simulink model "iwave_dsa_1ant"  (R2019a)
settings: Solver=VariableStepAuto  StartTime=0.0  StopTime=10.0  RelTol=1e-3
undefined symbols (not defined in the file): i
libraries: xbsIndex_r4 x9262, casper_library_misc x249, xps_library x3, casper_library_reorder x2, casper_library_delays x2
(part 32 of 96)

== system iwave_dsa_1ant/pipeline0/input/bit_stats/histogram ==
  note: pulse extend allows
      | input to AND gate at
      | t + 2^bitwidth + 1
  note: write on t+8, t+9
  note: input valid t+7, t+8
  note: addr presented here
      | t+5, t+6
  note: high t+4, t+5
  note: goes high
      | t+4
  note: new_acc goes high
      | at time t
  note: goes to zero
      | at t + 1
  note: 2^bitwidth extend
      | output goes low
      | at t+(2^bitwidth) + 1
  note: addr input to bram
      | t+6, t+7
  note: capture data 2 of 4 clocks,
      | starting two clocks after new_acc
  note: write on t+8, t+9
  note: goes to zero
      | at t + 1
  note: goes high at
      | at t + 2
  din : Inport
  new_acc : Inport  Port=2
  AddSub1 : xbsIndex_r4/AddSub  mode=Addition  use_carryin=off  use_carryout=off  en=off  latency=1  precision=User Defined  arith_type=Unsigned  n_bits=16  bin_pt=0  quantization=Truncate  overflow=Wrap  use_behavioral_HDL=on  hw_selection=Fabric  pipelined=off  dbl_ovrd=off  block_type=addsub
  AddSub2 : xbsIndex_r4/AddSub  mode=Addition  use_carryin=off  use_carryout=off  en=off  latency=1  precision=User Defined  arith_type=Unsigned  n_bits=16  bin_pt=0  quantization=Truncate  overflow=Wrap  use_behavioral_HDL=on  hw_selection=Fabric  pipelined=off  dbl_ovrd=off  block_type=addsub
  Concat : xbsIndex_r4/Concat  num_inputs=2  dbl_ovrd=off  block_type=concat
  Concat1 : xbsIndex_r4/Concat  num_inputs=2  dbl_ovrd=off  block_type=concat
  Constant1 : xbsIndex_r4/Constant  const=1  gui_display_data_type=Fixed-point  arith_type=Unsigned  n_bits=2  bin_pt=0  preci_type=Single  exp_width=8  frac_width=24  explicit_period=on  period=1  equ=P=C  opselect=C  inp2=PCIN>>17  opr=+  inp1=P  carry=CIN  dbl_ovrd=off  block_type=constant
  Constant2 : xbsIndex_r4/Constant  const=1  gui_display_data_type=Fixed-point  arith_type=Unsigned  n_bits=2  bin_pt=0  preci_type=Single  exp_width=8  frac_width=24  explicit_period=on  period=1  equ=P=C  opselect=C  inp2=PCIN>>17  opr=+  inp1=P  carry=CIN  dbl_ovrd=off  block_type=constant
  Constant3 : xbsIndex_r4/Constant  const=2  gui_display_data_type=Fixed-point  arith_type=Unsigned  n_bits=2  bin_pt=0  preci_type=Single  exp_width=8  frac_width=24  explicit_period=on  period=1  equ=P=C  opselect=C  inp2=PCIN>>17  opr=+  inp1=P  carry=CIN  dbl_ovrd=off  block_type=constant
  Constant4 : xbsIndex_r4/Constant  const=2  gui_display_data_type=Fixed-point  arith_type=Unsigned  n_bits=2  bin_pt=0  preci_type=Single  exp_width=8  frac_width=24  explicit_period=on  period=1  equ=P=C  opselect=C  inp2=PCIN>>17  opr=+  inp1=P  carry=CIN  dbl_ovrd=off  block_type=constant
  Constant5 : xbsIndex_r4/Constant  const=0  gui_display_data_type=Fixed-point  arith_type=Unsigned  n_bits=16  bin_pt=0  preci_type=Single  exp_width=8  frac_width=24  explicit_period=on  period=1  equ=P=C  opselect=C  inp2=PCIN>>17  opr=+  inp1=P  carry=CIN  dbl_ovrd=off  block_type=constant
  Constant6 : xbsIndex_r4/Constant  const=0  gui_display_data_type=Fixed-point  arith_type=Unsigned  n_bits=16  bin_pt=0  preci_type=Single  exp_width=8  frac_width=24  explicit_period=on  period=1  equ=P=C  opselect=C  inp2=PCIN>>17  opr=+  inp1=P  carry=CIN  dbl_ovrd=off  block_type=constant
  Constant7 : xbsIndex_r4/Constant  const=0  gui_display_data_type=Fixed-point  arith_type=Unsigned  n_bits=1  bin_pt=0  preci_type=Single  exp_width=8  frac_width=24  explicit_period=on  period=1  equ=P=C  opselect=C  inp2=PCIN>>17  opr=+  inp1=P  carry=CIN  dbl_ovrd=off  block_type=constant
  Constant8 : xbsIndex_r4/Constant  const=1  gui_display_data_type=Fixed-point  arith_type=Unsigned  n_bits=1  bin_pt=0  preci_type=Single  exp_width=8  frac_width=24  explicit_period=on  period=1  equ=P=C  opselect=C  inp2=PCIN>>17  opr=+  inp1=P  carry=CIN  dbl_ovrd=off  block_type=constant
  Counter1 : xbsIndex_r4/Counter  cnt_type=Free Running  cnt_to=Inf  operation=Up  start_count=0  cnt_by_val=1  arith_type=Unsigned  n_bits=2  bin_pt=0  load_pin=off  rst=on  en=off  explicit_period=on  period=1  use_behavioral_HDL=off  implementation=Fabric  dbl_ovrd=off  block_type=counter
  Counter3 : xbsIndex_r4/Counter  cnt_type=Free Running  cnt_to=Inf  operation=Up  start_count=0  cnt_by_val=1  arith_type=Unsigned  n_bits=bitwidth  bin_pt=0  load_pin=off  rst=off  en=off  explicit_period=on  period=1  use_behavioral_HDL=off  implementation=Fabric  dbl_ovrd=off  block_type=counter
  Counter4 : xbsIndex_r4/Counter  cnt_type=Free Running  cnt_to=Inf  operation=Up  start_count=0  cnt_by_val=1  arith_type=Unsigned  n_bits=2  bin_pt=0  load_pin=off  rst=on  en=off  explicit_period=on  period=1  use_behavioral_HDL=off  implementation=Fabric  dbl_ovrd=off  block_type=counter
  Delay{1..3,5,7..11,13,16..18,20..21,25..27} (18 alike) : xbsIndex_r4/Delay  rst=off  infoeditControl=Selection of Reset will increase slice count due to use of real FFs and instead of SRLs  en=off  latency=1  reg_retiming=off  dbl_ovrd=off  block_type=delay
  Delay{6,12,19,22} (4 alike) : xbsIndex_r4/Delay  rst=off  infoeditControl=Selection of Reset will increase slice count due to use of real FFs and instead of SRLs  en=off  latency=2  reg_retiming=off  dbl_ovrd=off  block_type=delay
  Delay{4,14..15,23} (4 alike) : xbsIndex_r4/Delay  rst=off  infoeditControl=Selection of Reset will increase slice count due to use of real FFs and instead of SRLs  en=off  latency=3  reg_retiming=off  dbl_ovrd=off  block_type=delay
  Delay24 : xbsIndex_r4/Delay  rst=off  infoeditControl=Selection of Reset will increase slice count due to use of real FFs and instead of SRLs  en=off  latency=2^bitwidth  reg_retiming=off  dbl_ovrd=off  block_type=delay
  Delay28 : xbsIndex_r4/Delay  rst=off  infoeditControl=Selection of Reset will increase slice count due to use of real FFs and instead of SRLs  en=off  latency=2^bitwidth  reg_retiming=off  dbl_ovrd=off  block_type=delay
  Delay29 : xbsIndex_r4/Delay  rst=off  infoeditControl=Selection of Reset will increase slice count due to use of real FFs and instead of SRLs  en=off  latency=2^bitwidth  reg_retiming=off  dbl_ovrd=off  block_type=delay
  Gateway Out{1..6} (6 alike) : xbsIndex_r4/Gateway Out  inherit_from_input=off  hdl_port=off  rows=1  columns=1  UseAsDAC=off  DACChannel='1'  interface=None  automatic_assignment=on  address_offset=hex2dec('00')  intf_name=''  intf_description=''  timing_constraint=None  locs_specified=off  LOCs={}  io_standard={}  block_type=gatewayout
  Inverter{,1..4} (5 alike) : xbsIndex_r4/Inverter  en=off  latency=0  dbl_ovrd=off  block_type=inv
  Logical{,2,5,7} (4 alike) : xbsIndex_r4/Logical  logical_function=AND  inputs=2  en=off  latency=1  precision=Full  arith_type=Unsigned  n_bits=16  bin_pt=0  align_bp=on  dbl_ovrd=off  block_type=logical
  Logical{1,3..4,6} (4 alike) : xbsIndex_r4/Logical  logical_function=AND  inputs=2  en=off  latency=0  precision=Full  arith_type=Unsigned  n_bits=16  bin_pt=0  align_bp=on  dbl_ovrd=off  block_type=logical
  Logical8 : xbsIndex_r4/Logical  logical_function=OR  inputs=2  en=off  latency=1  precision=Full  arith_type=Unsigned  n_bits=16  bin_pt=0  align_bp=on  dbl_ovrd=off  block_type=logical
  Mux{,1..5} (6 alike) : xbsIndex_r4/Mux  inputs=2  en=off  latency=1  precision=Full  arith_type=Unsigned  n_bits=16  bin_pt=14  quantization=Truncate  overflow=Wrap  dbl_ovrd=off  block_type=mux
  Register : xbsIndex_r4/Register  init=0  rst=off  en=on  dbl_ovrd=off  block_type=register
  Register1 : xbsIndex_r4/Register  init=0  rst=off  en=on  dbl_ovrd=off  block_type=register
  Relational : xbsIndex_r4/Relational  mode=a=b  op_type=Bool  en=off  latency=0  dbl_ovrd=off  block_type=relational
  Relational1 : xbsIndex_r4/Relational  mode=a=b  op_type=Bool  en=off  latency=0  dbl_ovrd=off  block_type=relational
  Slice : xbsIndex_r4/Slice  nbits=1  boolean_output=on  mode=Lower Bit Location + Width  bit1=0  base1=MSB of Input  bit0=1  base0=LSB of Input  dbl_ovrd=off  block_type=slice
  Slice1 : xbsIndex_r4/Slice  nbits=1  boolean_output=on  mode=Lower Bit Location + Width  bit1=0  base1=MSB of Input  bit0=1  base0=LSB of Input  dbl_ovrd=off  block_type=slice
  Terminator : Terminator
  To Workspace : ToWorkspace  VariableName=addr0  SaveFormat=Timeseries  SampleTime=-1
  To Workspace1 : ToWorkspace  VariableName=din0  SaveFormat=Timeseries  SampleTime=-1
  To Workspace2 : ToWorkspace  VariableName=en0  SaveFormat=Timeseries  SampleTime=-1
  To Workspace3 : ToWorkspace  VariableName=addr1  SaveFormat=Timeseries  SampleTime=-1
  To Workspace4 : ToWorkspace  VariableName=din1  SaveFormat=Timeseries  SampleTime=-1
  To Workspace5 : ToWorkspace  VariableName=en1  SaveFormat=Timeseries  SampleTime=-1
  output : Subsystem  Tag=xps:bram  AncestorBlock=xps_library/Memory/shared_bram  mask{sample_rate=1, init_vals=[0:2^10-1], data_bin_pt=0, optimization=Minimum_Area, reg_core_output=off, reg_prim_output=off, data_width=16, addr_width=bitwidth+1, arith_type=Unsigned, desc_str=|, type_desc=uint16}
      mask desc_str=|
      | BRAM storing histogram data. Word ``n`` in the
      | bottom half of the RAM stores the number of
      | occurances of of ADC sample code ``n`` in _even_
      | numbered ADC samples. Word ``n`` in the _top_
      | half of the RAM stores the number of occurances of
      | ADC sample code ``n`` in _odd_ numbered ADC
      | samples.
      mask prompts: sample_rate "Sample rate"; init_vals "Initial values (simulation only)"; data_bin_pt "Data Binary Point"; reg_core_output "Register Core Output"; reg_prim_output "Register Primitive Output"; data_width "Data Width"; addr_width "Address width"; arith_type "Output Data Type"; desc_str "Description"; type_desc "Word Type Description"
      mask init:
      | shared_bram_mask;
      mask TypeOptions optimization: Minimum_Area | Low_Power
      mask TypeOptions data_width: 8 | 16 | 32 | 64 | 128
      mask TypeOptions arith_type: Unsigned | Signed  (2's comp)
      mask DialogControl Container4 Prompt: Configuration
      mask DialogControl Container10 Prompt: Documentation
  pulse_ext : Subsystem  AncestorBlock=casper_library_misc/pulse_ext  mask(pulse_ext){pulse_len=2^bitwidth}
      mask prompts: pulse_len "Length of Pulse"
      mask help:
      | Extends a boolean signal to be high for the specified number of clocks after
      | the last high input.
      mask init:
      | bits = ceil(log2(pulse_len+1));
      mask Help: eval('xlWeb(''http://casper.berkeley.edu/wiki/Pulse_ext'')')
  ram0 : xbsIndex_r4/Dual Port RAM  depth=2^bitwidth  initVector=sin(pi*(0:15)/16)  distributed_mem=Block RAM  init_a=0  init_b=0  rst_a=off  rst_b=off  en_a=off  en_b=off  latency=1  write_mode_A=Read After Write  write_mode_B=Read Before Write  optimize=Area  dbl_ovrd=off  block_type=dpram
  ram1 : xbsIndex_r4/Dual Port RAM  depth=2^bitwidth  initVector=sin(pi*(0:15)/16)  distributed_mem=Block RAM  init_a=0  init_b=0  rst_a=off  rst_b=off  en_a=off  en_b=off  latency=1  write_mode_A=Read After Write  write_mode_B=Read Before Write  optimize=Area  dbl_ovrd=off  block_type=dpram
  wires:
  new_acc/1 -> Counter4/1, Counter1/1, pulse_ext/1(in)
  Inverter/1 -> Logical/2
  pulse_ext/1(out) -> Delay25/1, Inverter3/1, Delay9/1, Inverter/1
  Slice/1 -> Logical/1
  Logical/1 -> Delay21/1, Register/2, Logical2/1, Delay13/1
  Delay8/1 -> Delay15/1
  Delay9/1 -> Delay8/1
  Delay2/1 -> Concat/2, Gateway Out6/1
  Delay3/1 -> Logical8/1, Gateway Out1/1
  Gateway Out5/1 -> To Workspace3/1
  Gateway Out4/1 -> To Workspace4/1
  Gateway Out3/1 -> To Workspace5/1
  output/1(data_out) -> Terminator/1
  Gateway Out1/1 -> To Workspace2/1
  Gateway Out2/1 -> To Workspace1/1
  Gateway Out6/1 -> To Workspace/1
  Delay15/1 -> ram0/6, Delay3/1, Inverter1/1
  Counter1/1 -> Slice/1
  Delay17/1 -> Relational/2
  Mux1/1 -> ram0/1
  Constant2/1 -> Mux/2
  Constant3/1 -> Mux/3
  AddSub1/1 -> ram0/2
  ram0/1 -> AddSub1/1
  Mux/1 -> Delay20/1
  Delay20/1 -> AddSub1/2
  Delay19/1 -> Mux1/3
  Register/1 -> Mux1/2, Relational/1, Delay17/1, Delay19/1
  Delay22/1 -> Mux1/1
  Constant5/1 -> ram0/5
  ram0/2 -> Mux4/2, Gateway Out2/1
  Logical1/1 -> ram0/3
  Delay23/1 -> Logical1/1
  Inverter1/1 -> Logical1/2
  Delay21/1 -> Delay23/1, Delay22/1
  Delay7/1 -> Register/1
  Delay13/1 -> Logical2/2
  Relational/1 -> Logical3/1
  Logical3/1 -> Mux/1
  Logical2/1 -> Logical3/2
  Logical7/1 -> Delay11/1, Logical5/1, Delay1/1, Register1/2
  Delay16/1 -> Delay4/1
  Delay25/1 -> Delay16/1
  Delay4/1 -> Delay27/1, ram1/6, Inverter2/1
  Delay5/1 -> Relational1/2
  Mux3/1 -> ram1/1
  Constant1/1 -> Mux2/2
  Constant4/1 -> Mux2/3
  AddSub2/1 -> ram1/2
  ram1/1 -> AddSub2/1
  Mux2/1 -> Delay10/1
  Delay10/1 -> AddSub2/2
  Delay6/1 -> Mux3/3
  Register1/1 -> Mux3/2, Relational1/1, Delay5/1, Delay6/1
  Delay12/1 -> Mux3/1
  Constant6/1 -> ram1/5
  ram1/2 -> Delay24/1, Gateway Out4/1
  Logical4/1 -> ram1/3
  Delay14/1 -> Logical4/1
  Inverter2/1 -> Logical4/2
  Delay11/1 -> Delay14/1, Delay12/1
  Delay1/1 -> Logical5/2
  Relational1/1 -> Logical6/1
  Logical6/1 -> Mux2/1
  Logical5/1 -> Logical6/2
  Inverter3/1 -> Logical7/2
  Counter4/1 -> Slice1/1
  Slice1/1 -> Inverter4/1
  Inverter4/1 -> Logical7/1
  Delay18/1 -> Register1/1
  din/1 -> Delay18/1, Delay7/1
  Delay26/1 -> Delay29/1, Gateway Out5/1
  Mux4/1 -> output/2(data_in)
  Counter3/1 -> Delay2/1, ram1/4, Delay26/1, ram0/4
  Mux5/1 -> output/1(addr)
  Logical8/1 -> output/3(we)
  Delay27/1 -> Delay28/1, Gateway Out3/1
  Delay28/1 -> Mux5/1, Mux4/1, Logical8/2
  Delay24/1 -> Mux4/3
  Concat/1 -> Mux5/2
  Concat1/1 -> Mux5/3
  Delay29/1 -> Concat1/2
  Constant7/1 -> Concat/1
  Constant8/1 -> Concat1/1

== system iwave_dsa_1ant/pipeline0/input/bit_stats/input_sel ==
  sim_1 : Inport
  adm_pcie_9h7_dts_dual_2x100g_dsp_3b_pipeline0_input_bit_stats_input_sel_user_data_out : xbsIndex_r4/Gateway In  gui_display_data_type=Fixed-point  arith_type=Unsigned  n_bits=32  bin_pt=0  preci_type=Single  exp_width=8  frac_width=24  rows=1  columns=1  quantization="Round  (unbiased: +/- Inf)"  overflow=Saturate  period=1  UseAsADC=off  ADCChannel='1'  interface=None  automatic_assignment=on  address_offset=hex2dec('00')  intf_name=''  intf_description=''  default_value=0  timing_constraint=None  locs_specified=off  LOCs={}  io_standard={}  inherit_from_input=off  hdl_port=on  dbl_ovrd=off  block_type=gatewayin
  convert1_1 : DataTypeConversion  OutDataTypeStr=fixdt('ufix32_En0')  LockScale=on
  convert2_1 : DataTypeConversion  OutDataTypeStr=fixdt('ufix32_En0')  ConvertRealWorld=Stored Integer (SI)  LockScale=on
  gain_1 : Gain
  io_delay : xbsIndex_r4/Delay  rst=off  infoeditControl=Selection of Reset will increase slice count due to use of real FFs and instead of SRLs  en=off  latency=0  reg_retiming=on  dbl_ovrd=off  block_type=delay
  reint1 : xbsIndex_r4/Reinterpret  force_arith_type=on  arith_type=Unsigned  force_bin_pt=on  bin_pt=0  block_type=reinterpret
  slice_reg : xbsIndex_r4/Slice  nbits=32  boolean_output=off  mode=Lower Bit Location + Width  bit1=0  base1=MSB of Input  bit0=0  base0=LSB of Input  dbl_ovrd=off  block_type=slice
  in_reg : Outport
  wires:
  adm_pcie_9h7_dts_dual_2x100g_dsp_3b_pipeline0_input_bit_stats_input_sel_user_data_out/1 -> io_delay/1
  sim_1/1 -> convert1_1/1
  convert1_1/1 -> convert2_1/1
  convert2_1/1 -> gain_1/1
  gain_1/1 -> adm_pcie_9h7_dts_dual_2x100g_dsp_3b_pipeline0_input_bit_stats_input_sel_user_data_out/1
  io_delay/1 -> slice_reg/1
  slice_reg/1 -> reint1/1
  reint1/1 -> in_reg/1

== system iwave_dsa_1ant/pipeline0/input/bus_mux/d_bussify ==
  in1 : Inport
  in2 : Inport  Port=2
  in3 : Inport  Port=3
  in4 : Inport  Port=4
  concatenate : xbsIndex_r4/Concat  num_inputs=4  dbl_ovrd=off  block_type=concat
  reinterpret{1..4} (4 alike) : xbsIndex_r4/Reinterpret  force_arith_type=on  arith_type=Unsigned  force_bin_pt=on  bin_pt=0  block_type=reinterpret
      reinterpret1 settings: infoedit="Changes signal type without altering the binary representation.   You can changed the signal between signed and unsigned, and relocate the binary point.<br><br>Hardware notes: In hardware this block costs nothing.<br><br>Example:  Suppose the input is 6 bits wide, signed, with 2 fractional bits, and the output is forced to unsigned with 0 fractional bits.  Then an input of -2.0 (1110.00 in binary 2's complement) becomes an output of 56 (111000 in binary)."
      reinterpret2 settings: infoedit="Changes signal type without altering the binary representation.   You can changed the signal between signed and unsigned, and relocate the binary point.<br><br>Hardware notes: In hardware this block costs nothing.<br><br>Example:  Suppose the input is 6 bits wide, signed, with 2 fractional bits, and the output is forced to unsigned with 0 fractional bits.  Then an input of -2.0 (1110.00 in binary 2's complement) becomes an output of 56 (111000 in binary)."
  bus_out : Outport
  wires:
  concatenate/1 -> bus_out/1
  in1/1 -> reinterpret1/1
  reinterpret1/1 -> concatenate/1
  in2/1 -> reinterpret2/1
  reinterpret2/1 -> concatenate/2
  in3/1 -> reinterpret3/1
  reinterpret3/1 -> concatenate/3
  in4/1 -> reinterpret4/1
  reinterpret4/1 -> concatenate/4

== system iwave_dsa_1ant/pipeline0/input/bus_mux/expand0 ==
  bus_in : Inport
  reinterpret{1..4} (4 alike) : xbsIndex_r4/Reinterpret  force_arith_type=on  arith_type=Unsigned  force_bin_pt=on  bin_pt=0  block_type=reinterpret
  slice1 : xbsIndex_r4/Slice  nbits=192  boolean_output=off  mode=Upper Bit Location + Width  bit1=-576  base1=MSB of Input  bit0=0  base0=LSB of Input  dbl_ovrd=off  block_type=slice
  slice2 : xbsIndex_r4/Slice  nbits=192  boolean_output=off  mode=Upper Bit Location + Width  bit1=-384  base1=MSB of Input  bit0=0  base0=LSB of Input  dbl_ovrd=off  block_type=slice
  slice3 : xbsIndex_r4/Slice  nbits=192  boolean_output=off  mode=Upper Bit Location + Width  bit1=-192  base1=MSB of Input  bit0=0  base0=LSB of Input  dbl_ovrd=off  block_type=slice
  slice4 : xbsIndex_r4/Slice  nbits=192  boolean_output=off  mode=Upper Bit Location + Width  bit1=0  base1=MSB of Input  bit0=0  base0=LSB of Input  dbl_ovrd=off  block_type=slice
  msb_out4 : Outport
  out3 : Outport  Port=2
  out2 : Outport  Port=3
  lsb_out1 : Outport  Port=4
  wires:
  bus_in/1 -> slice4/1, slice3/1, slice2/1, slice1/1
  slice4/1 -> reinterpret4/1
  reinterpret4/1 -> msb_out4/1
  slice3/1 -> reinterpret3/1
  reinterpret3/1 -> out3/1
  slice2/1 -> reinterpret2/1
  reinterpret2/1 -> out2/1
  slice1/1 -> reinterpret1/1
  reinterpret1/1 -> lsb_out1/1

== system iwave_dsa_1ant/pipeline0/input/bus_mux/expand1 ==
  bus_in : Inport
  reinterpret{1..4} (4 alike) : xbsIndex_r4/Reinterpret  force_arith_type=on  arith_type=Unsigned  force_bin_pt=on  bin_pt=0  block_type=reinterpret
  slice1 : xbsIndex_r4/Slice  nbits=192  boolean_output=off  mode=Upper Bit Location + Width  bit1=-576  base1=MSB of Input  bit0=0  base0=LSB of Input  dbl_ovrd=off  block_type=slice
  slice2 : xbsIndex_r4/Slice  nbits=192  boolean_output=off  mode=Upper Bit Location + Width  bit1=-384  base1=MSB of Input  bit0=0  base0=LSB of Input  dbl_ovrd=off  block_type=slice
  slice3 : xbsIndex_r4/Slice  nbits=192  boolean_output=off  mode=Upper Bit Location + Width  bit1=-192  base1=MSB of Input  bit0=0  base0=LSB of Input  dbl_ovrd=off  block_type=slice
  slice4 : xbsIndex_r4/Slice  nbits=192  boolean_output=off  mode=Upper Bit Location + Width  bit1=0  base1=MSB of Input  bit0=0  base0=LSB of Input  dbl_ovrd=off  block_type=slice
  msb_out4 : Outport
  out3 : Outport  Port=2
  out2 : Outport  Port=3
  lsb_out1 : Outport  Port=4
  wires:
  bus_in/1 -> slice4/1, slice3/1, slice2/1, slice1/1
  slice4/1 -> reinterpret4/1
  reinterpret4/1 -> msb_out4/1
  slice3/1 -> reinterpret3/1
  reinterpret3/1 -> out3/1
  slice2/1 -> reinterpret2/1
  reinterpret2/1 -> out2/1
  slice1/1 -> reinterpret1/1
  reinterpret1/1 -> lsb_out1/1

== system iwave_dsa_1ant/pipeline0/input/bus_mux/expand2 ==
  bus_in : Inport
  reinterpret{1..4} (4 alike) : xbsIndex_r4/Reinterpret  force_arith_type=on  arith_type=Unsigned  force_bin_pt=on  bin_pt=0  block_type=reinterpret
  slice1 : xbsIndex_r4/Slice  nbits=192  boolean_output=off  mode=Upper Bit Location + Width  bit1=-576  base1=MSB of Input  bit0=0  base0=LSB of Input  dbl_ovrd=off  block_type=slice
  slice2 : xbsIndex_r4/Slice  nbits=192  boolean_output=off  mode=Upper Bit Location + Width  bit1=-384  base1=MSB of Input  bit0=0  base0=LSB of Input  dbl_ovrd=off  block_type=slice
  slice3 : xbsIndex_r4/Slice  nbits=192  boolean_output=off  mode=Upper Bit Location + Width  bit1=-192  base1=MSB of Input  bit0=0  base0=LSB of Input  dbl_ovrd=off  block_type=slice
  slice4 : xbsIndex_r4/Slice  nbits=192  boolean_output=off  mode=Upper Bit Location + Width  bit1=0  base1=MSB of Input  bit0=0  base0=LSB of Input  dbl_ovrd=off  block_type=slice
  msb_out4 : Outport
  out3 : Outport  Port=2
  out2 : Outport  Port=3
  lsb_out1 : Outport  Port=4
  wires:
  bus_in/1 -> slice4/1, slice3/1, slice2/1, slice1/1
  slice4/1 -> reinterpret4/1
  reinterpret4/1 -> msb_out4/1
  slice3/1 -> reinterpret3/1
  reinterpret3/1 -> out3/1
  slice2/1 -> reinterpret2/1
  reinterpret2/1 -> out2/1
  slice1/1 -> reinterpret1/1
  reinterpret1/1 -> lsb_out1/1

== system iwave_dsa_1ant/pipeline0/input/bus_mux/sel_expand ==
  bus_in : Inport
  reinterpret{1..4} (4 alike) : xbsIndex_r4/Reinterpret  force_arith_type=on  arith_type=Unsigned  force_bin_pt=on  bin_pt=0  block_type=reinterpret
  slice1 : xbsIndex_r4/Slice  nbits=2  boolean_output=off  mode=Upper Bit Location + Width  bit1=-6  base1=MSB of Input  bit0=0  base0=LSB of Input  dbl_ovrd=off  block_type=slice
  slice2 : xbsIndex_r4/Slice  nbits=2  boolean_output=off  mode=Upper Bit Location + Width  bit1=-4  base1=MSB of Input  bit0=0  base0=LSB of Input  dbl_ovrd=off  block_type=slice
  slice3 : xbsIndex_r4/Slice  nbits=2  boolean_output=off  mode=Upper Bit Location + Width  bit1=-2  base1=MSB of Input  bit0=0  base0=LSB of Input  dbl_ovrd=off  block_type=slice
  slice4 : xbsIndex_r4/Slice  nbits=2  boolean_output=off  mode=Upper Bit Location + Width  bit1=0  base1=MSB of Input  bit0=0  base0=LSB of Input  dbl_ovrd=off  block_type=slice
  msb_out4 : Outport
  out3 : Outport  Port=2
  out2 : Outport  Port=3
  lsb_out1 : Outport  Port=4
  wires:
  bus_in/1 -> slice4/1, slice3/1, slice2/1, slice1/1
  slice4/1 -> reinterpret4/1
  reinterpret4/1 -> msb_out4/1
  slice3/1 -> reinterpret3/1
  reinterpret3/1 -> out3/1
  slice2/1 -> reinterpret2/1
  reinterpret2/1 -> out2/1
  slice1/1 -> reinterpret1/1
  reinterpret1/1 -> lsb_out1/1

== system iwave_dsa_1ant/pipeline0/input/rms/Subsystem ==
  In1 : Inport
  In2 : Inport  Port=2
  In3 : Inport  Port=3
  In4 : Inport  Port=4
  In5 : Inport  Port=5
  In6 : Inport  Port=6
  In7 : Inport  Port=7
  In8 : Inport  Port=8
  In9 : Inport  Port=9
  In10 : Inport  Port=10
  In11 : Inport  Port=11
  In12 : Inport  Port=12
  In13 : Inport  Port=13
  In14 : Inport  Port=14
  In15 : Inport  Port=15
  In16 : Inport  Port=16
  In17 : Inport  Port=17
  In18 : Inport  Port=18
  In19 : Inport  Port=19
  In20 : Inport  Port=20
  In21 : Inport  Port=21
  In22 : Inport  Port=22
  In23 : Inport  Port=23
  In24 : Inport  Port=24
  In25 : Inport  Port=25
  In26 : Inport  Port=26
  In27 : Inport  Port=27
  In28 : Inport  Port=28
  In29 : Inport  Port=29
  In30 : Inport  Port=30
  In31 : Inport  Port=31
  In32 : Inport  Port=32
  calc_adc_sum_sq0 : Subsystem
  calc_adc_sum_sq1 : Subsystem
  calc_adc_sum_sq10 : Subsystem
  calc_adc_sum_sq11 : Subsystem
  calc_adc_sum_sq12 : Subsystem
  calc_adc_sum_sq13 : Subsystem
  calc_adc_sum_sq14 : Subsystem
  calc_adc_sum_sq15 : Subsystem
  calc_adc_sum_sq16 : Subsystem
  calc_adc_sum_sq17 : Subsystem
  calc_adc_sum_sq18 : Subsystem
  calc_adc_sum_sq19 : Subsystem
  calc_adc_sum_sq2 : Subsystem
  calc_adc_sum_sq20 : Subsystem
  calc_adc_sum_sq21 : Subsystem
  calc_adc_sum_sq22 : Subsystem
  calc_adc_sum_sq23 : Subsystem
  calc_adc_sum_sq24 : Subsystem
  calc_adc_sum_sq25 : Subsystem
  calc_adc_sum_sq26 : Subsystem
  calc_adc_sum_sq27 : Subsystem
  calc_adc_sum_sq28 : Subsystem
  calc_adc_sum_sq29 : Subsystem
  calc_adc_sum_sq3 : Subsystem
  calc_adc_sum_sq30 : Subsystem
  calc_adc_sum_sq31 : Subsystem
  calc_adc_sum_sq4 : Subsystem
  calc_adc_sum_sq5 : Subsystem
  calc_adc_sum_sq6 : Subsystem
  calc_adc_sum_sq7 : Subsystem
  calc_adc_sum_sq8 : Subsystem
  calc_adc_sum_sq9 : Subsystem
  Out1 : Outport
  Out2 : Outport  Port=2
  Out3 : Outport  Port=3
  Out4 : Outport  Port=4
  Out5 : Outport  Port=5
  Out6 : Outport  Port=6
  Out7 : Outport  Port=7
  Out8 : Outport  Port=8
  Out9 : Outport  Port=9
  Out10 : Outport  Port=10
  Out11 : Outport  Port=11
  Out12 : Outport  Port=12
  Out13 : Outport  Port=13
  Out14 : Outport  Port=14
  Out15 : Outport  Port=15
  Out16 : Outport  Port=16
  Out17 : Outport  Port=17
  Out18 : Outport  Port=18
  Out19 : Outport  Port=19
  Out20 : Outport  Port=20
  Out21 : Outport  Port=21
  Out22 : Outport  Port=22
  Out23 : Outport  Port=23
  Out24 : Outport  Port=24
  Out25 : Outport  Port=25
  Out26 : Outport  Port=26
  Out27 : Outport  Port=27
  Out28 : Outport  Port=28
  Out29 : Outport  Port=29
  Out30 : Outport  Port=30
  Out31 : Outport  Port=31
  Out32 : Outport  Port=32
  wires:
  calc_adc_sum_sq19/1(sum_sumsq) -> Out28/1
  In30/1 -> calc_adc_sum_sq21/1(in)
  calc_adc_sum_sq0/1(sum_sumsq) -> Out1/1
  In18/1 -> calc_adc_sum_sq17/1(in)
  calc_adc_sum_sq18/1(sum_sumsq) -> Out27/1
  calc_adc_sum_sq4/1(sum_sumsq) -> Out5/1
  In4/1 -> calc_adc_sum_sq3/1(in)
  In20/1 -> calc_adc_sum_sq25/1(in)
  calc_adc_sum_sq3/1(sum_sumsq) -> Out4/1
  calc_adc_sum_sq12/1(sum_sumsq) -> Out13/1
  In12/1 -> calc_adc_sum_sq11/1(in)
  In28/1 -> calc_adc_sum_sq19/1(in)
  calc_adc_sum_sq20/1(sum_sumsq) -> Out29/1
  calc_adc_sum_sq24/1(sum_sumsq) -> Out19/1
  In10/1 -> calc_adc_sum_sq9/1(in)
  In14/1 -> calc_adc_sum_sq13/1(in)
  calc_adc_sum_sq23/1(sum_sumsq) -> Out32/1
  calc_adc_sum_sq6/1(sum_sumsq) -> Out7/1
  calc_adc_sum_sq25/1(sum_sumsq) -> Out20/1
  In25/1 -> calc_adc_sum_sq30/1(in)
  calc_adc_sum_sq13/1(sum_sumsq) -> Out14/1
  In27/1 -> calc_adc_sum_sq18/1(in)
  In19/1 -> calc_adc_sum_sq24/1(in)
  In13/1 -> calc_adc_sum_sq12/1(in)
  In15/1 -> calc_adc_sum_sq14/1(in)
  calc_adc_sum_sq15/1(sum_sumsq) -> Out16/1
  calc_adc_sum_sq28/1(sum_sumsq) -> Out23/1
  calc_adc_sum_sq2/1(sum_sumsq) -> Out3/1
  In1/1 -> calc_adc_sum_sq0/1(in)
  calc_adc_sum_sq17/1(sum_sumsq) -> Out18/1
  In5/1 -> calc_adc_sum_sq4/1(in)
  In16/1 -> calc_adc_sum_sq15/1(in)
  calc_adc_sum_sq10/1(sum_sumsq) -> Out11/1
  calc_adc_sum_sq22/1(sum_sumsq) -> Out31/1
  In21/1 -> calc_adc_sum_sq26/1(in)
  In11/1 -> calc_adc_sum_sq10/1(in)
  In22/1 -> calc_adc_sum_sq27/1(in)
  In32/1 -> calc_adc_sum_sq23/1(in)
  In29/1 -> calc_adc_sum_sq20/1(in)
  In7/1 -> calc_adc_sum_sq6/1(in)
  calc_adc_sum_sq1/1(sum_sumsq) -> Out2/1
  In3/1 -> calc_adc_sum_sq2/1(in)
  calc_adc_sum_sq16/1(sum_sumsq) -> Out17/1
  In24/1 -> calc_adc_sum_sq29/1(in)
  calc_adc_sum_sq27/1(sum_sumsq) -> Out22/1
  In23/1 -> calc_adc_sum_sq28/1(in)
  calc_adc_sum_sq11/1(sum_sumsq) -> Out12/1
  calc_adc_sum_sq31/1(sum_sumsq) -> Out26/1
  calc_adc_sum_sq26/1(sum_sumsq) -> Out21/1
  calc_adc_sum_sq30/1(sum_sumsq) -> Out25/1
  calc_adc_sum_sq21/1(sum_sumsq) -> Out30/1
  In2/1 -> calc_adc_sum_sq1/1(in)
  calc_adc_sum_sq29/1(sum_sumsq) -> Out24/1
  calc_adc_sum_sq8/1(sum_sumsq) -> Out9/1
  calc_adc_sum_sq7/1(sum_sumsq) -> Out8/1
  calc_adc_sum_sq14/1(sum_sumsq) -> Out15/1
  In9/1 -> calc_adc_sum_sq8/1(in)
  In31/1 -> calc_adc_sum_sq22/1(in)
  In8/1 -> calc_adc_sum_sq7/1(in)
  In26/1 -> calc_adc_sum_sq31/1(in)
  calc_adc_sum_sq5/1(sum_sumsq) -> Out6/1
  In6/1 -> calc_adc_sum_sq5/1(in)
  In17/1 -> calc_adc_sum_sq16/1(in)
  calc_adc_sum_sq9/1(sum_sumsq) -> Out10/1

== system iwave_dsa_1ant/pipeline0/input/rms/Subsystem1 ==
  In1 : Inport
  In2 : Inport  Port=2
  In3 : Inport  Port=3
  In4 : Inport  Port=4
  In5 : Inport  Port=5
  In6 : Inport  Port=6
  In7 : Inport  Port=7
  In8 : Inport  Port=8
  In9 : Inport  Port=9
  In10 : Inport  Port=10
  In11 : Inport  Port=11
  In12 : Inport  Port=12
  In13 : Inport  Port=13
  In14 : Inport  Port=14
  In15 : Inport  Port=15
  In16 : Inport  Port=16
  In17 : Inport  Port=17
  In18 : Inport  Port=18
  In19 : Inport  Port=19
  In20 : Inport  Port=20
  In21 : Inport  Port=21
  In22 : Inport  Port=22
  In23 : Inport  Port=23
  In24 : Inport  Port=24
  In25 : Inport  Port=25
  In26 : Inport  Port=26
  In27 : Inport  Port=27
  In28 : Inport  Port=28
  In29 : Inport  Port=29
  In30 : Inport  Port=30
  In31 : Inport  Port=31
  In32 : Inport  Port=32
  calc_adc_sum_sq0 : Subsystem
  calc_adc_sum_sq1 : Subsystem
  calc_adc_sum_sq10 : Subsystem
  calc_adc_sum_sq11 : Subsystem
  calc_adc_sum_sq12 : Subsystem
  calc_adc_sum_sq13 : Subsystem
  calc_adc_sum_sq14 : Subsystem
  calc_adc_sum_sq15 : Subsystem
  calc_adc_sum_sq16 : Subsystem
  calc_adc_sum_sq17 : Subsystem
  calc_adc_sum_sq18 : Subsystem
  calc_adc_sum_sq19 : Subsystem
  calc_adc_sum_sq2 : Subsystem
  calc_adc_sum_sq20 : Subsystem
  calc_adc_sum_sq21 : Subsystem
  calc_adc_sum_sq22 : Subsystem
  calc_adc_sum_sq23 : Subsystem
  calc_adc_sum_sq24 : Subsystem
  calc_adc_sum_sq25 : Subsystem
  calc_adc_sum_sq26 : Subsystem
  calc_adc_sum_sq27 : Subsystem
  calc_adc_sum_sq28 : Subsystem
  calc_adc_sum_sq29 : Subsystem
  calc_adc_sum_sq3 : Subsystem
  calc_adc_sum_sq30 : Subsystem
  calc_adc_sum_sq31 : Subsystem
  calc_adc_sum_sq4 : Subsystem
  calc_adc_sum_sq5 : Subsystem
  calc_adc_sum_sq6 : Subsystem
  calc_adc_sum_sq7 : Subsystem
  calc_adc_sum_sq8 : Subsystem
  calc_adc_sum_sq9 : Subsystem
  Out1 : Outport
  Out2 : Outport  Port=2
  Out3 : Outport  Port=3
  Out4 : Outport  Port=4
  Out5 : Outport  Port=5
  Out6 : Outport  Port=6
  Out7 : Outport  Port=7
  Out8 : Outport  Port=8
  Out9 : Outport  Port=9
  Out10 : Outport  Port=10
  Out11 : Outport  Port=11
  Out12 : Outport  Port=12
  Out13 : Outport  Port=13
  Out14 : Outport  Port=14
  Out15 : Outport  Port=15
  Out16 : Outport  Port=16
  Out17 : Outport  Port=17
  Out18 : Outport  Port=18
  Out19 : Outport  Port=19
  Out20 : Outport  Port=20
  Out21 : Outport  Port=21
  Out22 : Outport  Port=22
  Out23 : Outport  Port=23
  Out24 : Outport  Port=24
  Out25 : Outport  Port=25
  Out26 : Outport  Port=26
  Out27 : Outport  Port=27
  Out28 : Outport  Port=28
  Out29 : Outport  Port=29
  Out30 : Outport  Port=30
  Out31 : Outport  Port=31
  Out32 : Outport  Port=32
  wires:
  calc_adc_sum_sq9/1(sum_sumsq) -> Out10/1
  In17/1 -> calc_adc_sum_sq16/1(in)
  In6/1 -> calc_adc_sum_sq5/1(in)
  calc_adc_sum_sq5/1(sum_sumsq) -> Out6/1
  In26/1 -> calc_adc_sum_sq31/1(in)
  In8/1 -> calc_adc_sum_sq7/1(in)
  In31/1 -> calc_adc_sum_sq22/1(in)
  In9/1 -> calc_adc_sum_sq8/1(in)
  calc_adc_sum_sq14/1(sum_sumsq) -> Out15/1
  calc_adc_sum_sq7/1(sum_sumsq) -> Out8/1
  calc_adc_sum_sq8/1(sum_sumsq) -> Out9/1
  calc_adc_sum_sq29/1(sum_sumsq) -> Out24/1
  In2/1 -> calc_adc_sum_sq1/1(in)
  calc_adc_sum_sq21/1(sum_sumsq) -> Out30/1
  calc_adc_sum_sq30/1(sum_sumsq) -> Out25/1
  calc_adc_sum_sq26/1(sum_sumsq) -> Out21/1
  calc_adc_sum_sq31/1(sum_sumsq) -> Out26/1
  calc_adc_sum_sq11/1(sum_sumsq) -> Out12/1
  In23/1 -> calc_adc_sum_sq28/1(in)
  calc_adc_sum_sq27/1(sum_sumsq) -> Out22/1
  In24/1 -> calc_adc_sum_sq29/1(in)
  calc_adc_sum_sq16/1(sum_sumsq) -> Out17/1
  In3/1 -> calc_adc_sum_sq2/1(in)
  calc_adc_sum_sq1/1(sum_sumsq) -> Out2/1
  In7/1 -> calc_adc_sum_sq6/1(in)
  In29/1 -> calc_adc_sum_sq20/1(in)
  In32/1 -> calc_adc_sum_sq23/1(in)
  In22/1 -> calc_adc_sum_sq27/1(in)
  In11/1 -> calc_adc_sum_sq10/1(in)
  In21/1 -> calc_adc_sum_sq26/1(in)
  calc_adc_sum_sq22/1(sum_sumsq) -> Out31/1
  calc_adc_sum_sq10/1(sum_sumsq) -> Out11/1
  In16/1 -> calc_adc_sum_sq15/1(in)
  In5/1 -> calc_adc_sum_sq4/1(in)
  calc_adc_sum_sq17/1(sum_sumsq) -> Out18/1
  In1/1 -> calc_adc_sum_sq0/1(in)
  calc_adc_sum_sq2/1(sum_sumsq) -> Out3/1
  calc_adc_sum_sq28/1(sum_sumsq) -> Out23/1
  calc_adc_sum_sq15/1(sum_sumsq) -> Out16/1
  In15/1 -> calc_adc_sum_sq14/1(in)
  In13/1 -> calc_adc_sum_sq12/1(in)
  In19/1 -> calc_adc_sum_sq24/1(in)
  In27/1 -> calc_adc_sum_sq18/1(in)
  calc_adc_sum_sq13/1(sum_sumsq) -> Out14/1
  In25/1 -> calc_adc_sum_sq30/1(in)
  calc_adc_sum_sq25/1(sum_sumsq) -> Out20/1
  calc_adc_sum_sq6/1(sum_sumsq) -> Out7/1
  calc_adc_sum_sq23/1(sum_sumsq) -> Out32/1
  In14/1 -> calc_adc_sum_sq13/1(in)
  In10/1 -> calc_adc_sum_sq9/1(in)
  calc_adc_sum_sq24/1(sum_sumsq) -> Out19/1
  calc_adc_sum_sq20/1(sum_sumsq) -> Out29/1
  In28/1 -> calc_adc_sum_sq19/1(in)
  In12/1 -> calc_adc_sum_sq11/1(in)
  calc_adc_sum_sq12/1(sum_sumsq) -> Out13/1
  calc_adc_sum_sq3/1(sum_sumsq) -> Out4/1
  In20/1 -> calc_adc_sum_sq25/1(in)
  In4/1 -> calc_adc_sum_sq3/1(in)
  calc_adc_sum_sq4/1(sum_sumsq) -> Out5/1
  calc_adc_sum_sq18/1(sum_sumsq) -> Out27/1
  In18/1 -> calc_adc_sum_sq17/1(in)
  calc_adc_sum_sq0/1(sum_sumsq) -> Out1/1
  In30/1 -> calc_adc_sum_sq21/1(in)
  calc_adc_sum_sq19/1(sum_sumsq) -> Out28/1

== system iwave_dsa_1ant/pipeline0/input/rms/Subsystem2 ==
  In1 : Inport
  In2 : Inport  Port=2
  In3 : Inport  Port=3
  In4 : Inport  Port=4
  In5 : Inport  Port=5
  In6 : Inport  Port=6
  In7 : Inport  Port=7
  In8 : Inport  Port=8
  In9 : Inport  Port=9
  In10 : Inport  Port=10
  In11 : Inport  Port=11
  In12 : Inport  Port=12
  In13 : Inport  Port=13
  In14 : Inport  Port=14
  In15 : Inport  Port=15
  In16 : Inport  Port=16
  In17 : Inport  Port=17
  In18 : Inport  Port=18
  In19 : Inport  Port=19
  In20 : Inport  Port=20
  In21 : Inport  Port=21
  In22 : Inport  Port=22
  In23 : Inport  Port=23
  In24 : Inport  Port=24
  In25 : Inport  Port=25
  In26 : Inport  Port=26
  In27 : Inport  Port=27
  In28 : Inport  Port=28
  In29 : Inport  Port=29
  In30 : Inport  Port=30
  In31 : Inport  Port=31
  In32 : Inport  Port=32
  calc_adc_sum_sq0 : Subsystem
  calc_adc_sum_sq1 : Subsystem
  calc_adc_sum_sq10 : Subsystem
  calc_adc_sum_sq11 : Subsystem
  calc_adc_sum_sq12 : Subsystem
  calc_adc_sum_sq13 : Subsystem
  calc_adc_sum_sq14 : Subsystem
  calc_adc_sum_sq15 : Subsystem
  calc_adc_sum_sq16 : Subsystem
  calc_adc_sum_sq17 : Subsystem
  calc_adc_sum_sq18 : Subsystem
  calc_adc_sum_sq19 : Subsystem
  calc_adc_sum_sq2 : Subsystem
  calc_adc_sum_sq20 : Subsystem
  calc_adc_sum_sq21 : Subsystem
  calc_adc_sum_sq22 : Subsystem
  calc_adc_sum_sq23 : Subsystem
  calc_adc_sum_sq24 : Subsystem
  calc_adc_sum_sq25 : Subsystem
  calc_adc_sum_sq26 : Subsystem
  calc_adc_sum_sq27 : Subsystem
  calc_adc_sum_sq28 : Subsystem
  calc_adc_sum_sq29 : Subsystem
  calc_adc_sum_sq3 : Subsystem
  calc_adc_sum_sq30 : Subsystem
  calc_adc_sum_sq31 : Subsystem
  calc_adc_sum_sq4 : Subsystem
  calc_adc_sum_sq5 : Subsystem
  calc_adc_sum_sq6 : Subsystem
  calc_adc_sum_sq7 : Subsystem
  calc_adc_sum_sq8 : Subsystem
  calc_adc_sum_sq9 : Subsystem
  Out1 : Outport
  Out2 : Outport  Port=2
  Out3 : Outport  Port=3
  Out4 : Outport  Port=4
  Out5 : Outport  Port=5
  Out6 : Outport  Port=6
  Out7 : Outport  Port=7
  Out8 : Outport  Port=8
  Out9 : Outport  Port=9
  Out10 : Outport  Port=10
  Out11 : Outport  Port=11
  Out12 : Outport  Port=12
  Out13 : Outport  Port=13
  Out14 : Outport  Port=14
  Out15 : Outport  Port=15
  Out16 : Outport  Port=16
  Out17 : Outport  Port=17
  Out18 : Outport  Port=18
  Out19 : Outport  Port=19
  Out20 : Outport  Port=20
  Out21 : Outport  Port=21
  Out22 : Outport  Port=22
  Out23 : Outport  Port=23
  Out24 : Outport  Port=24
  Out25 : Outport  Port=25
  Out26 : Outport  Port=26
  Out27 : Outport  Port=27
  Out28 : Outport  Port=28
  Out29 : Outport  Port=29
  Out30 : Outport  Port=30
  Out31 : Outport  Port=31
  Out32 : Outport  Port=32
  wires:
  calc_adc_sum_sq19/1(sum_sumsq) -> Out28/1
  In30/1 -> calc_adc_sum_sq21/1(in)
  calc_adc_sum_sq0/1(sum_sumsq) -> Out1/1
  In18/1 -> calc_adc_sum_sq17/1(in)
  calc_adc_sum_sq18/1(sum_sumsq) -> Out27/1
  calc_adc_sum_sq4/1(sum_sumsq) -> Out5/1
  In4/1 -> calc_adc_sum_sq3/1(in)
  In20/1 -> calc_adc_sum_sq25/1(in)
  calc_adc_sum_sq3/1(sum_sumsq) -> Out4/1
  calc_adc_sum_sq12/1(sum_sumsq) -> Out13/1
  In12/1 -> calc_adc_sum_sq11/1(in)
  In28/1 -> calc_adc_sum_sq19/1(in)
  calc_adc_sum_sq20/1(sum_sumsq) -> Out29/1
  calc_adc_sum_sq24/1(sum_sumsq) -> Out19/1
  In10/1 -> calc_adc_sum_sq9/1(in)
  In14/1 -> calc_adc_sum_sq13/1(in)
  calc_adc_sum_sq23/1(sum_sumsq) -> Out32/1
  calc_adc_sum_sq6/1(sum_sumsq) -> Out7/1
  calc_adc_sum_sq25/1(sum_sumsq) -> Out20/1
  In25/1 -> calc_adc_sum_sq30/1(in)
  calc_adc_sum_sq13/1(sum_sumsq) -> Out14/1
  In27/1 -> calc_adc_sum_sq18/1(in)
  In19/1 -> calc_adc_sum_sq24/1(in)
  In13/1 -> calc_adc_sum_sq12/1(in)
  In15/1 -> calc_adc_sum_sq14/1(in)
  calc_adc_sum_sq15/1(sum_sumsq) -> Out16/1
  calc_adc_sum_sq28/1(sum_sumsq) -> Out23/1
  calc_adc_sum_sq2/1(sum_sumsq) -> Out3/1
  In1/1 -> calc_adc_sum_sq0/1(in)
  calc_adc_sum_sq17/1(sum_sumsq) -> Out18/1
  In5/1 -> calc_adc_sum_sq4/1(in)
  In16/1 -> calc_adc_sum_sq15/1(in)
  calc_adc_sum_sq10/1(sum_sumsq) -> Out11/1
  calc_adc_sum_sq22/1(sum_sumsq) -> Out31/1
  In21/1 -> calc_adc_sum_sq26/1(in)
  In11/1 -> calc_adc_sum_sq10/1(in)
  In22/1 -> calc_adc_sum_sq27/1(in)
  In32/1 -> calc_adc_sum_sq23/1(in)
  In29/1 -> calc_adc_sum_sq20/1(in)
  In7/1 -> calc_adc_sum_sq6/1(in)
  calc_adc_sum_sq1/1(sum_sumsq) -> Out2/1
  In3/1 -> calc_adc_sum_sq2/1(in)
  calc_adc_sum_sq16/1(sum_sumsq) -> Out17/1
  In24/1 -> calc_adc_sum_sq29/1(in)
  calc_adc_sum_sq27/1(sum_sumsq) -> Out22/1
  In23/1 -> calc_adc_sum_sq28/1(in)
  calc_adc_sum_sq11/1(sum_sumsq) -> Out12/1
  calc_adc_sum_sq31/1(sum_sumsq) -> Out26/1
  calc_adc_sum_sq26/1(sum_sumsq) -> Out21/1
  calc_adc_sum_sq30/1(sum_sumsq) -> Out25/1
  calc_adc_sum_sq21/1(sum_sumsq) -> Out30/1
  In2/1 -> calc_adc_sum_sq1/1(in)
  calc_adc_sum_sq29/1(sum_sumsq) -> Out24/1
  calc_adc_sum_sq8/1(sum_sumsq) -> Out9/1
  calc_adc_sum_sq7/1(sum_sumsq) -> Out8/1
  calc_adc_sum_sq14/1(sum_sumsq) -> Out15/1
  In9/1 -> calc_adc_sum_sq8/1(in)
  In31/1 -> calc_adc_sum_sq22/1(in)
  In8/1 -> calc_adc_sum_sq7/1(in)
  In26/1 -> calc_adc_sum_sq31/1(in)
  calc_adc_sum_sq5/1(sum_sumsq) -> Out6/1
  In6/1 -> calc_adc_sum_sq5/1(in)
  In17/1 -> calc_adc_sum_sq16/1(in)
  calc_adc_sum_sq9/1(sum_sumsq) -> Out10/1

== system iwave_dsa_1ant/pipeline0/input/rms/Subsystem3 ==
  In1 : Inport
  In2 : Inport  Port=2
  In3 : Inport  Port=3
  In4 : Inport  Port=4
  In5 : Inport  Port=5
  In6 : Inport  Port=6
  In7 : Inport  Port=7
  In8 : Inport  Port=8
  In9 : Inport  Port=9
  In10 : Inport  Port=10
  In11 : Inport  Port=11
  In12 : Inport  Port=12
  In13 : Inport  Port=13
  In14 : Inport  Port=14
  In15 : Inport  Port=15
  In16 : Inport  Port=16
  In17 : Inport  Port=17
  In18 : Inport  Port=18
  In19 : Inport  Port=19
  In20 : Inport  Port=20
  In21 : Inport  Port=21
  In22 : Inport  Port=22
  In23 : Inport  Port=23
  In24 : Inport  Port=24
  In25 : Inport  Port=25
  In26 : Inport  Port=26
  In27 : Inport  Port=27
  In28 : Inport  Port=28
  In29 : Inport  Port=29
  In30 : Inport  Port=30
  In31 : Inport  Port=31
  In32 : Inport  Port=32
  calc_adc_sum_sq0 : Subsystem
  calc_adc_sum_sq1 : Subsystem
  calc_adc_sum_sq10 : Subsystem
  calc_adc_sum_sq11 : Subsystem
  calc_adc_sum_sq12 : Subsystem
  calc_adc_sum_sq13 : Subsystem
  calc_adc_sum_sq14 : Subsystem
  calc_adc_sum_sq15 : Subsystem
  calc_adc_sum_sq16 : Subsystem
  calc_adc_sum_sq17 : Subsystem
  calc_adc_sum_sq18 : Subsystem
  calc_adc_sum_sq19 : Subsystem
  calc_adc_sum_sq2 : Subsystem
  calc_adc_sum_sq20 : Subsystem
  calc_adc_sum_sq21 : Subsystem
  calc_adc_sum_sq22 : Subsystem
  calc_adc_sum_sq23 : Subsystem
  calc_adc_sum_sq24 : Subsystem
  calc_adc_sum_sq25 : Subsystem
  calc_adc_sum_sq26 : Subsystem
  calc_adc_sum_sq27 : Subsystem
  calc_adc_sum_sq28 : Subsystem
  calc_adc_sum_sq29 : Subsystem
  calc_adc_sum_sq3 : Subsystem
  calc_adc_sum_sq30 : Subsystem
  calc_adc_sum_sq31 : Subsystem
  calc_adc_sum_sq4 : Subsystem
  calc_adc_sum_sq5 : Subsystem
  calc_adc_sum_sq6 : Subsystem
  calc_adc_sum_sq7 : Subsystem
  calc_adc_sum_sq8 : Subsystem
  calc_adc_sum_sq9 : Subsystem
  Out1 : Outport
  Out2 : Outport  Port=2
  Out3 : Outport  Port=3
  Out4 : Outport  Port=4
  Out5 : Outport  Port=5
  Out6 : Outport  Port=6
  Out7 : Outport  Port=7
  Out8 : Outport  Port=8
  Out9 : Outport  Port=9
  Out10 : Outport  Port=10
  Out11 : Outport  Port=11
  Out12 : Outport  Port=12
  Out13 : Outport  Port=13
  Out14 : Outport  Port=14
  Out15 : Outport  Port=15
  Out16 : Outport  Port=16
  Out17 : Outport  Port=17
  Out18 : Outport  Port=18
  Out19 : Outport  Port=19
  Out20 : Outport  Port=20
  Out21 : Outport  Port=21
  Out22 : Outport  Port=22
  Out23 : Outport  Port=23
  Out24 : Outport  Port=24
  Out25 : Outport  Port=25
  Out26 : Outport  Port=26
  Out27 : Outport  Port=27
  Out28 : Outport  Port=28
  Out29 : Outport  Port=29
  Out30 : Outport  Port=30
  Out31 : Outport  Port=31
  Out32 : Outport  Port=32
  wires:
  calc_adc_sum_sq9/1(sum_sumsq) -> Out10/1
  In17/1 -> calc_adc_sum_sq16/1(in)
  In6/1 -> calc_adc_sum_sq5/1(in)
  calc_adc_sum_sq5/1(sum_sumsq) -> Out6/1
  In26/1 -> calc_adc_sum_sq31/1(in)
  In8/1 -> calc_adc_sum_sq7/1(in)
  In31/1 -> calc_adc_sum_sq22/1(in)
  In9/1 -> calc_adc_sum_sq8/1(in)
  calc_adc_sum_sq14/1(sum_sumsq) -> Out15/1
  calc_adc_sum_sq7/1(sum_sumsq) -> Out8/1
  calc_adc_sum_sq8/1(sum_sumsq) -> Out9/1
  calc_adc_sum_sq29/1(sum_sumsq) -> Out24/1
  In2/1 -> calc_adc_sum_sq1/1(in)
  calc_adc_sum_sq21/1(sum_sumsq) -> Out30/1
  calc_adc_sum_sq30/1(sum_sumsq) -> Out25/1
  calc_adc_sum_sq26/1(sum_sumsq) -> Out21/1
  calc_adc_sum_sq31/1(sum_sumsq) -> Out26/1
  calc_adc_sum_sq11/1(sum_sumsq) -> Out12/1
  In23/1 -> calc_adc_sum_sq28/1(in)
  calc_adc_sum_sq27/1(sum_sumsq) -> Out22/1
  In24/1 -> calc_adc_sum_sq29/1(in)
  calc_adc_sum_sq16/1(sum_sumsq) -> Out17/1
  In3/1 -> calc_adc_sum_sq2/1(in)
  calc_adc_sum_sq1/1(sum_sumsq) -> Out2/1
  In7/1 -> calc_adc_sum_sq6/1(in)
  In29/1 -> calc_adc_sum_sq20/1(in)
  In32/1 -> calc_adc_sum_sq23/1(in)
  In22/1 -> calc_adc_sum_sq27/1(in)
  In11/1 -> calc_adc_sum_sq10/1(in)
  In21/1 -> calc_adc_sum_sq26/1(in)
  calc_adc_sum_sq22/1(sum_sumsq) -> Out31/1
  calc_adc_sum_sq10/1(sum_sumsq) -> Out11/1
  In16/1 -> calc_adc_sum_sq15/1(in)
  In5/1 -> calc_adc_sum_sq4/1(in)
  calc_adc_sum_sq17/1(sum_sumsq) -> Out18/1
  In1/1 -> calc_adc_sum_sq0/1(in)
  calc_adc_sum_sq2/1(sum_sumsq) -> Out3/1
  calc_adc_sum_sq28/1(sum_sumsq) -> Out23/1
  calc_adc_sum_sq15/1(sum_sumsq) -> Out16/1
  In15/1 -> calc_adc_sum_sq14/1(in)
  In13/1 -> calc_adc_sum_sq12/1(in)
  In19/1 -> calc_adc_sum_sq24/1(in)
  In27/1 -> calc_adc_sum_sq18/1(in)
  calc_adc_sum_sq13/1(sum_sumsq) -> Out14/1
  In25/1 -> calc_adc_sum_sq30/1(in)
  calc_adc_sum_sq25/1(sum_sumsq) -> Out20/1
  calc_adc_sum_sq6/1(sum_sumsq) -> Out7/1
  calc_adc_sum_sq23/1(sum_sumsq) -> Out32/1
  In14/1 -> calc_adc_sum_sq13/1(in)
  In10/1 -> calc_adc_sum_sq9/1(in)
  calc_adc_sum_sq24/1(sum_sumsq) -> Out19/1
  calc_adc_sum_sq20/1(sum_sumsq) -> Out29/1
  In28/1 -> calc_adc_sum_sq19/1(in)
  In12/1 -> calc_adc_sum_sq11/1(in)
  calc_adc_sum_sq12/1(sum_sumsq) -> Out13/1
  calc_adc_sum_sq3/1(sum_sumsq) -> Out4/1
  In20/1 -> calc_adc_sum_sq25/1(in)
  In4/1 -> calc_adc_sum_sq3/1(in)
  calc_adc_sum_sq4/1(sum_sumsq) -> Out5/1
  calc_adc_sum_sq18/1(sum_sumsq) -> Out27/1
  In18/1 -> calc_adc_sum_sq17/1(in)
  calc_adc_sum_sq0/1(sum_sumsq) -> Out1/1
  In30/1 -> calc_adc_sum_sq21/1(in)
  calc_adc_sum_sq19/1(sum_sumsq) -> Out28/1
